simulink model "IPM_RotorPosition"  (R2022b)
settings: Solver=FixedStepAuto  StartTime=0.0  StopTime=Tsimulation  FixedStep=1e-4  RelTol=1e-4
values from neighbouring files (symbols this model uses):
  B = 0.05*Tn/Wm_n    (= 7.5e-05)    [Project_parameters.m]
  duty = T_pulse/Ts*100    (= 0.1)    [Project_parameters.m]
  J = 1e-4*1000000    (= 100)    [Project_parameters.m]
  Jload = 4*J    (= 400)    [Project_parameters.m]
  Lambda_mg = 0.252    [Project_parameters.m]
  Ld = 0.021    [Project_parameters.m]
  Lq = 0.128    [Project_parameters.m]
  p = 2    [Project_parameters.m]
  phase0 = 0    [Project_parameters.m]
  q = 4*In/2^10    (= 0.014765625)    [Project_parameters.m]
  R = 2.73    [Project_parameters.m]
  ramp = range/n_pulse/Ts    (= 0.157079632679)    [Project_parameters.m]
  theta0 = 28 * pi/180    (= 0.488692190558)    [Project_parameters.m]
  Ts = 1    [Project_parameters.m]
  U_pulse = 10    [Project_parameters.m]
libraries: simulink x1
settings Model: Creator=checc  LastModifiedBy=luca.salviato
settings SolverCC: AlgebraicLoopSolver=TrustRegion
settings DebuggingCC: UnconnectedInputMsg=warning  UnconnectedOutputMsg=warning  UnconnectedLineMsg=warning  SFMachineParentedDataDiag=warning
settings ModelReferenceCC: EnableRefExpFcnMdlSchedulingChecks=on

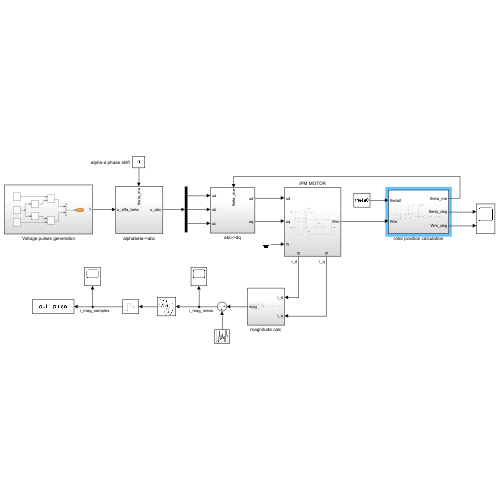
[thumbnail: Simulink's stored preview of the top-level diagram]
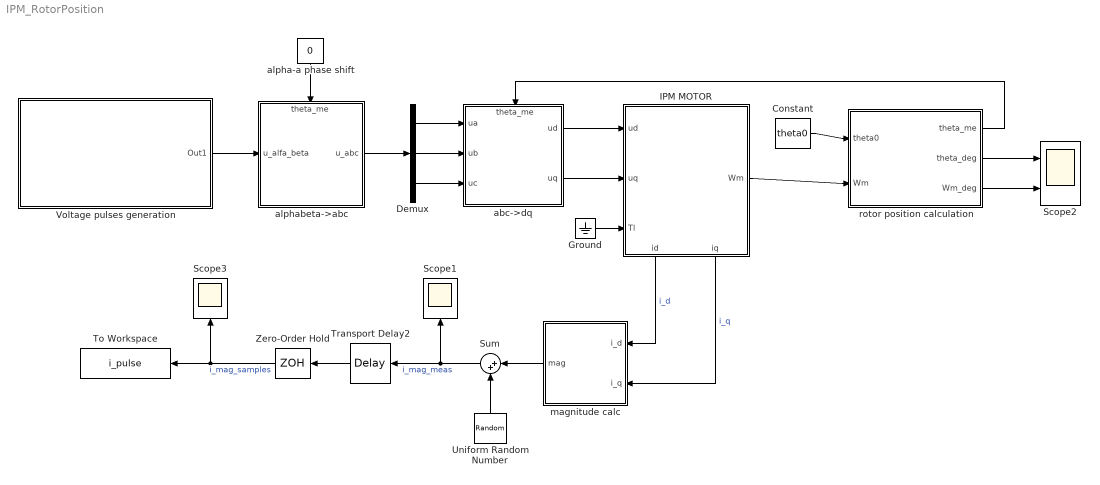
== system IPM_RotorPosition ==
  " alpha-a phase shift" : Constant  Value=0
  Constant : Constant  Value=theta0
  Demux : Demux  Outputs=3
  Ground : Ground
  IPM MOTOR : Subsystem
      settings: PortSchema="{\"entries\":[{\"content\":{\"sides\":[{\"content\":{\"connectorIds\":[\"In1\",\"In2\",\"In3\"]},\"type\":\"ConnectorPlacement.EquallySpacedRectSide\",\"uuid\":\"e30505c2-a625-46ad-8a51-33e67087bc0e\"},{\"content\":{\"connectorIds\":[\"Out1\"],\"side\":\"RIGHT\"},\"type\":\"ConnectorPlacement.EquallySpacedRectSide\",\"uuid\":\"a46b8d9d-4450-4313-b1e7-eed317c4b67c\"},{\"content\":{\"connectorIds\":[],\"side\":\"TOP\"},\"type\":\"ConnectorPlacement.EquallySpacedRectSide\",\"uuid\":\"a14c540d-7b37-4896-8aad-75427fdf86c4\"},{\"content\":{\"connectorIds\":[\"Out2\",\"Out3\"],\"side\":\"BOTTOM\"},\"type\":\"ConnectorPlacement.EquallySpacedRectSide\",\"uuid\":\"c12ebe95-0f8e-4a35-89aa-c6e50e57ad93\"}]},\"type\":\"ConnectorPlacement.EquallySpacedConnector\",\"uuid\":\"056724ea-377d-442e-a409-cafed055d923\"}],\"packageUris\":[\"http://schema.mathworks.com/mf0/Connector/R2020b\"],\"version\":\"1.0\"}"
  Scope1 : Scope
  Scope2 : Scope  NumInputPorts=2
  Scope3 : Scope
  Sum : Sum  Inputs=|++
  To Workspace : ToWorkspace  VariableName=i_pulse  SaveFormat=Timeseries  SampleTime=Ts
  Transport Delay2 : TransportDelay  DelayTime=Ts-duty*Ts/100
  Uniform Random Number : UniformRandomNumber  Minimum=-q/2  Maximum=q/2  SampleTime=0.1
  Voltage pulses generation : Subsystem
  Zero-Order Hold : ZeroOrderHold
  abc->dq : Subsystem
      settings: PortSchema="{\"entries\":[{\"content\":{\"sides\":[{\"content\":{\"connectorIds\":[\"In1\",\"In2\",\"In3\"]},\"type\":\"ConnectorPlacement.EquallySpacedRectSide\",\"uuid\":\"fe8e17e5-51f9-4d76-9762-24844d5591a5\"},{\"content\":{\"connectorIds\":[\"Out1\",\"Out2\"],\"side\":\"RIGHT\"},\"type\":\"ConnectorPlacement.EquallySpacedRectSide\",\"uuid\":\"fe87c28e-6767-4170-9643-60ca24f3ac9b\"},{\"content\":{\"connectorIds\":[\"In4\"],\"side\":\"TOP\"},\"type\":\"ConnectorPlacement.EquallySpacedRectSide\",\"uuid\":\"dea0d24c-4fb3-4d95-8bb7-9e0d73dd5c70\"},{\"content\":{\"connectorIds\":[],\"side\":\"BOTTOM\"},\"type\":\"ConnectorPlacement.EquallySpacedRectSide\",\"uuid\":\"c69c3b56-495d-4db3-bf8e-d9a29d84b68b\"}]},\"type\":\"ConnectorPlacement.EquallySpacedConnector\",\"uuid\":\"884fba33-6802-455d-a170-b85a256a9851\"}],\"packageUris\":[\"http://schema.mathworks.com/mf0/Connector/19700101\"],\"version\":\"1.0\"}"
  alphabeta->abc : Subsystem
      settings: PortSchema="{\"entries\":[{\"content\":{\"sides\":[{\"content\":{\"connectorIds\":[\"In1\"]},\"type\":\"ConnectorPlacement.EquallySpacedRectSide\",\"uuid\":\"4ffcad8d-ad4e-4b9f-9d99-70d9706481bd\"},{\"content\":{\"connectorIds\":[\"Out1\"],\"side\":\"RIGHT\"},\"type\":\"ConnectorPlacement.EquallySpacedRectSide\",\"uuid\":\"ca11e179-94fd-43b0-b2ab-d5b8ea31b40a\"},{\"content\":{\"connectorIds\":[\"In2\"],\"side\":\"TOP\"},\"type\":\"ConnectorPlacement.EquallySpacedRectSide\",\"uuid\":\"f9e7cc33-2dde-4aba-97f3-399a8c8ae3fe\"},{\"content\":{\"connectorIds\":[],\"side\":\"BOTTOM\"},\"type\":\"ConnectorPlacement.EquallySpacedRectSide\",\"uuid\":\"ae8b151b-7473-47fe-a384-ef12196a09bc\"}]},\"type\":\"ConnectorPlacement.EquallySpacedConnector\",\"uuid\":\"8c77ad63-71c2-4e35-a627-b120156b1a8b\"}],\"packageUris\":[\"http://schema.mathworks.com/mf0/Connector/19700101\"],\"version\":\"1.0\"}"
  magnitude calc : Subsystem
  rotor position calculation : Subsystem
  wires:
  abc->dq/1(ud) -> IPM MOTOR/1(ud)
  abc->dq/2(uq) -> IPM MOTOR/2(uq)
  Demux/1 -> abc->dq/1(ua)
  Demux/2 -> abc->dq/2(ub)
  Demux/3 -> abc->dq/3(uc)
  " alpha-a phase shift"/1 -> alphabeta->abc/2(theta_me)
  Sum/1 -> Transport Delay2/1, Scope1/1  "i_mag_meas"
  alphabeta->abc/1(u_abc) -> Demux/1
  Uniform Random Number/1 -> Sum/2
  Transport Delay2/1 -> Zero-Order Hold/1
  Zero-Order Hold/1 -> To Workspace/1, Scope3/1  "i_mag_samples"
  Voltage pulses generation/1(Out1) -> alphabeta->abc/1(u_alfa_beta)
  IPM MOTOR/2(id) -> magnitude calc/1(i_d)  "i_d"
  IPM MOTOR/3(iq) -> magnitude calc/2(i_q)  "i_q"
  magnitude calc/1(mag) -> Sum/1
  Constant/1 -> rotor position calculation/2(theta0)
  IPM MOTOR/1(Wm) -> rotor position calculation/1(Wm)
  rotor position calculation/2(theta_deg) -> Scope2/1
  rotor position calculation/1(Wm_deg) -> Scope2/2
  rotor position calculation/3(theta_me) -> abc->dq/4(theta_me)
  Ground/1 -> IPM MOTOR/3(Tl)

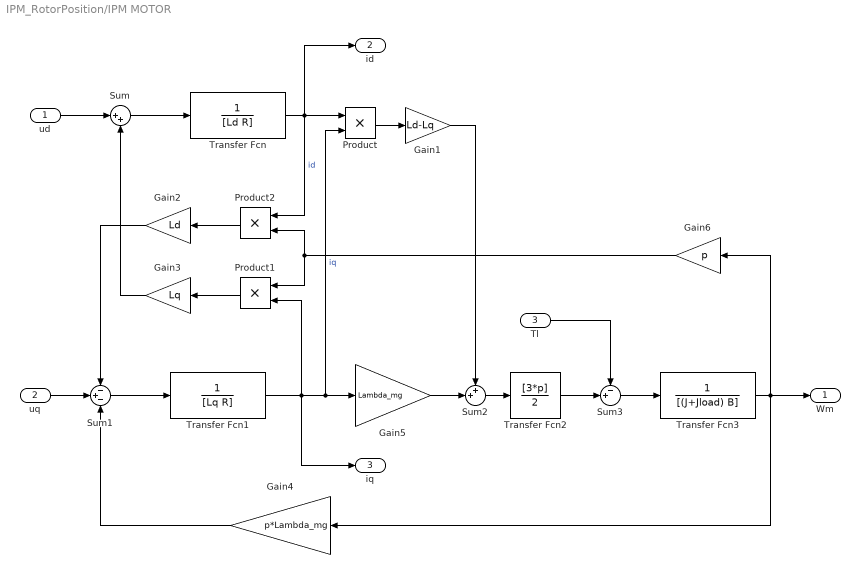
== system IPM_RotorPosition/IPM MOTOR ==
  ud : Inport
  uq : Inport  Port=2
  Tl : Inport  Port=3
  Gain1 : Gain  Gain=Ld-Lq
  Gain2 : Gain  Gain=Ld
  Gain3 : Gain  Gain=Lq
  Gain4 : Gain  Gain=p*Lambda_mg
  Gain5 : Gain  Gain=Lambda_mg
  Gain6 : Gain  Gain=p
  Product : Product
  Product1 : Product
  Product2 : Product
  Sum : Sum  Inputs=|++
  Sum1 : Sum  Inputs=-+-
  Sum2 : Sum  Inputs=++|
  Sum3 : Sum  Inputs=-+|
  Transfer Fcn : TransferFcn  Denominator=[Ld R]
  Transfer Fcn1 : TransferFcn  Denominator=[Lq R]
  Transfer Fcn2 : TransferFcn  Numerator=[3*p]  Denominator=[2]
  Transfer Fcn3 : TransferFcn  Denominator=[(J+Jload) B]
  Wm : Outport
  id : Outport  Port=2
  iq : Outport  Port=3
  wires:
  Transfer Fcn2/1 -> Sum3/2
  Gain1/1 -> Sum2/1
  Sum2/1 -> Transfer Fcn2/1
  Gain4/1 -> Sum1/3
  Gain5/1 -> Sum2/2
  Transfer Fcn1/1 -> Product1/2, Product/2, Gain5/1, iq/1  "iq"
  Product/1 -> Gain1/1
  Gain3/1 -> Sum/2
  Gain6/1 -> Product1/1, Product2/2
  uq/1 -> Sum1/2
  Gain2/1 -> Sum1/1
  Sum1/1 -> Transfer Fcn1/1
  Product1/1 -> Gain3/1
  Tl/1 -> Sum3/1
  Sum/1 -> Transfer Fcn/1
  Transfer Fcn3/1 -> Gain6/1, Gain4/1, Wm/1
  Product2/1 -> Gain2/1
  Transfer Fcn/1 -> Product2/1, Product/1, id/1  "id"
  ud/1 -> Sum/1
  Sum3/1 -> Transfer Fcn3/1

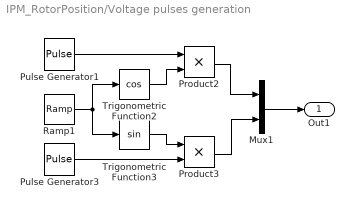
== system IPM_RotorPosition/Voltage pulses generation ==
  Mux1 : Mux  Inputs=2
  Product2 : Product
  Product3 : Product
  Pulse Generator1 : DiscretePulseGenerator  PulseType=Time based  Amplitude=U_pulse  Period=Ts  PulseWidth=duty
  Pulse Generator3 : DiscretePulseGenerator  PulseType=Time based  Amplitude=U_pulse  Period=Ts  PulseWidth=duty
  Ramp1 : simulink/Sources/Ramp  slope=ramp  start=0  InitialOutput=phase0
  Trigonometric Function2 : Trigonometry  Operator=cos
  Trigonometric Function3 : Trigonometry
  Out1 : Outport
  wires:
  Product2/1 -> Mux1/1
  Pulse Generator1/1 -> Product2/1
  Trigonometric Function3/1 -> Product3/1
  Pulse Generator3/1 -> Product3/2
  Trigonometric Function2/1 -> Product2/2
  Ramp1/1 -> Trigonometric Function3/1, Trigonometric Function2/1
  Product3/1 -> Mux1/2
  Mux1/1 -> Out1/1

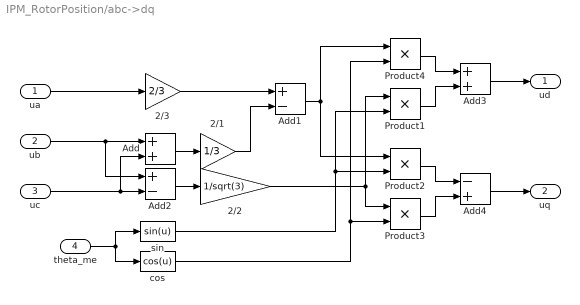
== system IPM_RotorPosition/abc->dq ==
  ua : Inport
  ub : Inport  Port=2
  uc : Inport  Port=3
  theta_me : Inport  Port=4
  2/1 : Gain  Gain=1/3  SaturateOnIntegerOverflow=on  OutDataTypeStr=Inherit: Same as input  ParamDataTypeStr=Inherit: Same as input
  2/2 : Gain  Gain=1/sqrt(3)  SaturateOnIntegerOverflow=on  OutDataTypeStr=Inherit: Same as input  ParamDataTypeStr=Inherit: Same as input
  2/3 : Gain  Gain=2/3  SaturateOnIntegerOverflow=on  OutDataTypeStr=Inherit: Same as input  ParamDataTypeStr=Inherit: Same as input
  Add : Sum
  Add1 : Sum  Inputs=+-
  Add2 : Sum  Inputs=+-
  Add3 : Sum
  Add4 : Sum  Inputs=-+
  Product{1..4} (4 alike) : Product  RndMeth=Zero
  cos : Fcn  Expr=cos(u)
  sin : Fcn  Expr=sin(u)
  ud : Outport
  uq : Outport  Port=2
  wires:
  ub/1 -> Add2/1, Add/1
  Add2/1 -> 2/2/1
  uc/1 -> Add2/2, Add/2
  2/3/1 -> Add1/1
  ua/1 -> 2/3/1
  2/1/1 -> Add1/2
  Add/1 -> 2/1/1
  theta_me/1 -> sin/1, cos/1
  Add1/1 -> Product2/1, Product4/1
  cos/1 -> Product3/2, Product4/2
  2/2/1 -> Product3/1, Product1/1
  sin/1 -> Product2/2, Product1/2
  Add3/1 -> ud/1
  Add4/1 -> uq/1
  Product4/1 -> Add3/1
  Product1/1 -> Add3/2
  Product2/1 -> Add4/1
  Product3/1 -> Add4/2

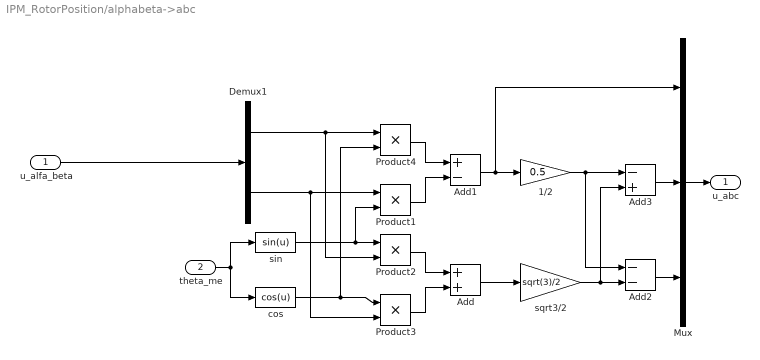
== system IPM_RotorPosition/alphabeta->abc ==
  u_alfa_beta : Inport
  theta_me : Inport  Port=2
  1/2 : Gain  Gain=0.5  SaturateOnIntegerOverflow=on  OutDataTypeStr=Inherit: Same as input  ParamDataTypeStr=Inherit: Same as input
  Add : Sum
  Add1 : Sum  Inputs=+-
  Add2 : Sum  Inputs=--
  Add3 : Sum  Inputs=-+
  Demux1 : Demux  Outputs=2
  Mux : Mux  Inputs=3
  Product{1..4} (4 alike) : Product  RndMeth=Zero
  cos : Fcn  Expr=cos(u)
  sin : Fcn  Expr=sin(u)
  sqrt3/2 : Gain  Gain=sqrt(3)/2  SaturateOnIntegerOverflow=on  OutDataTypeStr=Inherit: Same as input  ParamDataTypeStr=Inherit: Same as input
  u_abc : Outport
  wires:
  theta_me/1 -> sin/1, cos/1
  Demux1/1 -> Product4/1, Product2/2
  cos/1 -> Product4/2, Product3/1
  Demux1/2 -> Product1/1, Product3/2
  sin/1 -> Product1/2, Product2/1
  Product4/1 -> Add1/1
  Product1/1 -> Add1/2
  Product2/1 -> Add/1
  Product3/1 -> Add/2
  Add1/1 -> 1/2/1, Mux/1
  Add/1 -> sqrt3/2/1
  1/2/1 -> Add3/1, Add2/1
  sqrt3/2/1 -> Add3/2, Add2/2
  Add3/1 -> Mux/2
  Add2/1 -> Mux/3
  u_alfa_beta/1 -> Demux1/1
  Mux/1 -> u_abc/1

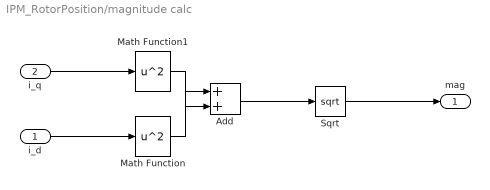
== system IPM_RotorPosition/magnitude calc ==
  i_d : Inport
  i_q : Inport  Port=2
  Add : Sum
  Math Function : Math  Operator=square
  Math Function1 : Math  Operator=square
  Sqrt : Sqrt
  mag : Outport
  wires:
  i_q/1 -> Math Function1/1
  Math Function1/1 -> Add/2
  Math Function/1 -> Add/1
  Sqrt/1 -> mag/1
  Add/1 -> Sqrt/1
  i_d/1 -> Math Function/1

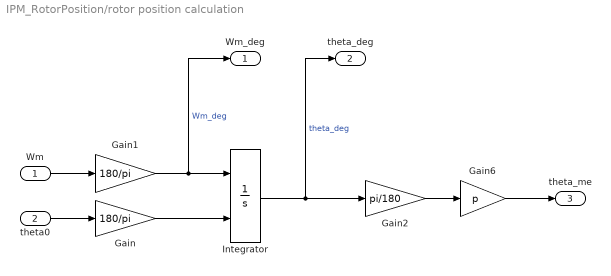
== system IPM_RotorPosition/rotor position calculation ==
  Wm : Inport
  theta0 : Inport  Port=2
  Gain : Gain  Gain=180/pi
  Gain1 : Gain  Gain=180/pi
  Gain2 : Gain  Gain=pi/180
  Gain6 : Gain  Gain=p
  Integrator : Integrator  InitialConditionSource=external
  Wm_deg : Outport
  theta_deg : Outport  Port=2
  theta_me : Outport  Port=3
  wires:
  Gain2/1 -> Gain6/1
  Integrator/1 -> Gain2/1, theta_deg/1  "theta_deg"
  Gain1/1 -> Wm_deg/1, Integrator/1  "Wm_deg"
  theta0/1 -> Gain/1
  Gain6/1 -> theta_me/1
  Gain/1 -> Integrator/2
  Wm/1 -> Gain1/1
